simulink subsystem "Inputs_Vehicle1D_Braking_refsub"  (R2026a)
settings: Solver=VariableStepAuto
libraries: simulink x1
settings Model: Creator=isaacito  LastModifiedBy=isaacito

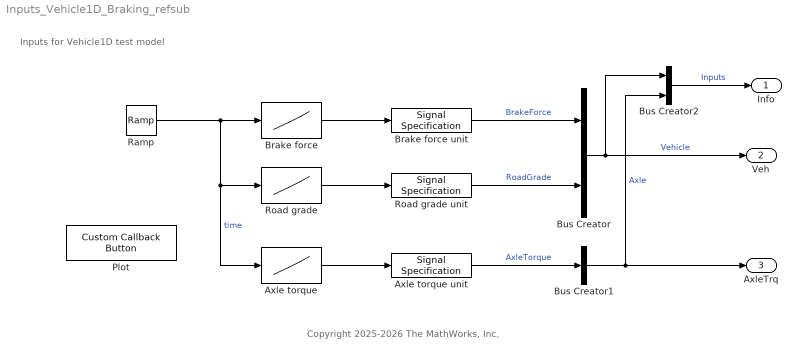
== system Inputs_Vehicle1D_Braking_refsub ==
  note: Inputs for Vehicle1D test model
  note: Copyright 2025-2026 The MathWorks, Inc.
  Axle torque : Lookup_n-D  NumberOfTableDimensions=1  BreakpointsForDimension1=[0; 5; 10]  Table=[0; 0; 0]  InterpMethod=Akima spline  InternalRulePriority=Speed  RndMeth=Simplest
  Axle torque unit : SignalSpecification  Unit=N*m
  Brake force : Lookup_n-D  NumberOfTableDimensions=1  BreakpointsForDimension1=[0; 50; 100; 103; 110; 155; 200; 205; 210; 255; 300; 370; 380; 390]  Table=[0; 0; 0; 3000; 0; 0; 0; 5000; 0; 0; 0; 3000; 3000; 3000]  InterpMethod=Akima spline  InternalRulePriority=Speed  RndMeth=Simplest
  Brake force unit : SignalSpecification  Unit=N
  Bus Creator : BusCreator  Inputs=2
  Bus Creator1 : BusCreator  Inputs=1
  Bus Creator2 : BusCreator  Inputs=2
  Plot : CustomCallbackButton  Configuration="{\"components\":[{\"name\":\"BackgroundImageComponent\",\"settings\":{\"image\":{\"size\":[0,0],\"src\":\"default\",\"srcOrientation\":\"Right\"},\"position\":[0,0,1,1]}},{\"name\":\"ButtonStateComponent\",\"settings\":{\"buttonType\":\"momentary\",\"clickFcn\":\"% Specify blocks to sort plot order.\\nblocks = [\\n  \\\"Brake force\\\"\\n  \\\"Road grade\\\"\\n  \\\"Axle torque\\\"\\n];\\nbev1mus.ModelUtil.plotLookupTable1DBlocks(gcs, Blocks=blocks, DivisionType=\\\"InterpolationInterval\\\", InterpolationInterval=0.1)\",\"onValue\":1,\"position\":[0,0,1,1],\"pressDelay\":\"500\",\"pressFcn\":\"\",\"repeatInterval\":\"0\",\"states\":[{\"horizontalAlignment\":\"center\",\"image\":{\"position\":[0,0,1,1],\"size\":[1,1],\"src\":\"default\",\"srcOrientation\":\"Right\"},\"label\":{\"color\":[0.01176470588,0.01176470588,0.01176470588,1],\"icon\":{\"size\":[0,0],\"src\":\"default\",\"srcOrientation\":\"Right\"},\"iconOffset\":0,\"iconPlacement\":\"left\",\"opacity\":1,\"show\":true,\"text\":{\"content\":\"Lookup tables\",\"font\":\"Helvetica\"}},\"labelOffset\":[0,0],\"verticalAlignment\":\"middle\"},{\"horizontalAlignment\":\"center\",\"image\":{\"position\":[0,0,1,1],\"size\":[1,1],\"src\":\"default\",\"srcOrientation\":\"Right\"},\"label\":{\"color\":[0.01176470588,0.01176470588,0.01176470588,1],\"icon\":{\"size\":[0,0],\"src\":\"default\",\"srcOrientation\":\"Right\"},\"iconOffset\":0,\"iconPlacement\":\"left\",\"opacity\":1,\"show\":true,\"text\":{\"content\":\"Lookup tables\",\"font\":\"Helvetica\"}},\"labelOffset\":[0,0],\"verticalAlignment\":\"middle\"},{\"horizontalAlignment\":\"center\",\"image\":{\"position\":[0,0,1,1],\"size\":[1,1],\"src\":\"default\",\"srcOrientation\":\"Right\"},\"label\":{\"color\":[0.01176470588,0.01176470588,0.01176470588,1],\"icon\":{\"size\":[0,0],\"src\":\"default\",\"srcOrientation\":\"Right\"},\"iconOffset\":0,\"iconPlacement\":\"left\",\"opacity\":1,\"show\":true,\"text\":{\"content\":\"Lookup tables\",\"font\":\"Helvetica\"}},\"labelOffset\":[0,0],\"verticalAlignment\":\"middle\"},{\"horizontalAlignment\":\"center\",\"image\":{\"position\":[0,0,1,1],\"size\":[1,1],\"src\":\"default\",\"srcOrientation\":\"Right\"},\"label\":{\"color\":[0.01176470588,0.01176470588,0.01176470588,1],\"icon\":{\"size\":[0,0],\"src\":\"default\",\"srcOrientation\":\"Right\"},\"iconOffset\":0,\"iconPlacement\":\"left\",\"opacity\":1,\"show\":true,\"text\":{\"content\":\"Lookup tables\",\"font\":\"Helvetica\"}},\"labelOffset\":[0,0],\"verticalAlignment\":\"middle\"}]}},{\"name\":\"ForegroundImageComponent\",\"settings\":{\"image\":{\"size\":[0,0],\"src\":\"default\",\"srcOrientation\":\"Right\"},\"isForeground\":1,\"position\":[0,0,1,1]}}],\"derived\":{\"blockParameters\":{\"AutoActivate\":true,\"ButtonText\":\"Lookup tables\",\"ButtonType\":\"Momentary\",\"ClickFcn\":\"% Specify blocks to sort plot order.\\nblocks = [\\n  \\\"Brake force\\\"\\n  \\\"Road grade\\\"\\n  \\\"Axle torque\\\"\\n];\\nbev1mus.ModelUtil.plotLookupTable1DBlocks(gcs, Blocks=blocks, DivisionType=\\\"InterpolationInterval\\\", InterpolationInterval=0.1)\",\"OnValue\":1,\"PressDelay\":\"500\",\"PressFcn\":\"\",\"RepeatInterval\":\"0\",\"fixedAspectRatio\":\"off\"}},\"settings\":{\"BindingType\":\"standalone\",\"autoActivate\":true,\"backgroundColor\":[244,244,244,1],\"backgroundOffset\":0.2,\"backgroundOpacity\":1,\"fixedAspectRatio\":\"off\",\"foregroundColor\":[0.01176470588,0.01176470588,0.01176470588,1],\"migratedFromLegacy\":true,\"useBackgroundColor\":true,\"variant\":\"callback\",\"version\":\"R2025a\"},\"type\":\"Button\"}"  CustomBackgroundColor="{\"color\":[0.9568627451,0.9568627451,0.9568627451],\"show\":true}"
  Ramp : simulink/Sources/Ramp  slope=1  start=0  InitialOutput=0
      settings: AttributesFormatString=|
      | Slope: %<slope>
      | Start time: %<start>
      | Initial output: %<InitialOutput>
  Road grade : Lookup_n-D  NumberOfTableDimensions=1  BreakpointsForDimension1=[0; 2.5; 5; 10; 255; 500; 520; 760; 1000]  Table=[0; 0; 0; -7; -7; -7; -4; -4; -4]  InterpMethod=Akima spline  InternalRulePriority=Speed  RndMeth=Simplest
  Road grade unit : SignalSpecification  Unit=%
  Info : Outport
  Veh : Outport  Port=2
  AxleTrq : Outport  Port=3  Unit=N*m
  wires:
  Bus Creator/1 -> Veh/1, Bus Creator2/1  "Vehicle"
  Brake force unit/1 -> Bus Creator/1  "BrakeForce"
  Road grade unit/1 -> Bus Creator/2  "RoadGrade"
  Axle torque unit/1 -> Bus Creator1/1  "AxleTorque"
  Bus Creator1/1 -> AxleTrq/1, Bus Creator2/2  "Axle"
  Bus Creator2/1 -> Info/1  "Inputs"
  Brake force/1 -> Brake force unit/1
  Road grade/1 -> Road grade unit/1
  Axle torque/1 -> Axle torque unit/1
  Ramp/1 -> Axle torque/1, Road grade/1, Brake force/1  "time"
